simulink model "robot_stand"  (R2014b)
settings: Solver=ode45  StartTime=0.0  StopTime=10  FixedStep=1e-4  RelTol=1e-3
values from neighbouring files (symbols this model uses):
  robot_floor_friction_coeff = 0.6    [robot_init.m]
  robot_floor_position_gain = -1e5    (= -100000)    [robot_init.m]
  robot_floor_speed_gain = -1e3    (= -1000)    [robot_init.m]
  robot_gravity = [0 0 -9.80665]    [robot_init.m]
undefined symbols (not defined in the file or in its folder): CM730_acc_center, CM730_acc_gain, CM730_default, CM730_gyro_center, CM730_gyro_gain, CM730_sample_time, FSR_max, FSR_no_load, FSR_sample_time, FSR_scale, MX28_default, MX28_inertia, MX28_Te, X, Y, Z
libraries: sm_lib x158, fl_lib x128, nesl_utility x77
(part 3 of 6)

== system robot_stand/Left Leg/Left Hip Pitch (12) ==
  Inertia : sm_lib/Body Elements/Inertia  InertiaType=Custom  Mass=1  MassUnits=g  CenterOfMass=[0 0 0]  CenterOfMassUnits=m  MomentsOfInertia=[0 0 MX28_inertia]  MomentsOfInertiaUnits=kg*m^2  ProductsOfInertia=[0 0 0]  ProductsOfInertiaUnits=kg*m^2  BlockFunction=simmechanics.library.body_elements.inertia
  MX28 Command : DataStoreRead  DataStoreName=MX28_ID12  SampleTime=MX28_Te  DataStoreElements=MX28_ID12.CW_angle_limit#MX28_ID12.CCW_angle_limit#MX28_ID12.torque_enable#MX28_ID12.D_gain#MX28_ID12.I_gain#MX28_ID12.P_gain#MX28_ID12.goal_position#MX28_ID12.moving_speed#MX28_ID12.torque_limit
  MX28 State : DataStoreWrite  DataStoreName=MX28_ID12  DataStoreElements=MX28_ID12.present_position#MX28_ID12.present_speed#MX28_ID12.present_load#MX28_ID12.moving#MX28_ID12.pwm
  Model : ModelReference  ModelNameDialog=MX28.slx  SimulationMode=Normal  ModelReferenceVersion=1.66  CopyOfModelName=MX28.slx  DefaultDataLogging=on
  Position converter : nesl_utility/PS-Simulink Converter  PhysicalDomain=network_engine_domain  SubClassName=ps_output  LeftPortType=input  RightPortType=output  PseudoPeriodic=off  Frequencies=[]  Unit=rad  AffineConversion=off
  Revolute Joint : sm_lib/Joints/Revolute Joint  SenseConstraintForce=off  SenseConstraintForceX=off  SenseConstraintForceY=off  SenseConstraintForceZ=off  SenseConstraintTorque=off  SenseConstraintTorqueX=off  SenseConstraintTorqueY=off  SenseConstraintTorqueZ=off  SenseTotalForce=off  SenseTotalForceX=off  SenseTotalForceY=off  SenseTotalForceZ=off  SenseTotalTorque=off  SenseTotalTorqueX=off  SenseTotalTorqueY=off  SenseTotalTorqueZ=off  CompositeWrenchDir=FollowerOnBase  CompositeWrenchFrame=BaseFrame  EquilibriumPosition=0  EquilibriumPositionUnits=deg  SpringStiffness=0  SpringStiffnessUnits=N*m/deg  DampingCoefficient=MX28_lub_friction  DampingCoefficientUnits=N*m/(rad/s)  TorqueActuationMode=InputTorque  MotionActuationMode=ComputedMotion  SensePosition=on  SenseVelocity=on  SenseAcceleration=off  SenseTorqueForce=off  PositionTargetValue=MX28_init_position  PositionTargetValueUnits=rad  PositionTargetSpecify=on  PositionTargetPriority=High  VelocityTargetValue=MX28_init_speed  VelocityTargetValueUnits=rad/s  VelocityTargetSpecify=on  VelocityTargetPriority=High  BlockFunction=simmechanics.library.joints.revolute_joint
  Speed converter : nesl_utility/PS-Simulink Converter  PhysicalDomain=network_engine_domain  SubClassName=ps_output  LeftPortType=input  RightPortType=output  PseudoPeriodic=off  Frequencies=[]  Unit=rad/s  AffineConversion=off
  Torque converter : nesl_utility/Simulink-PS Converter  PhysicalDomain=network_engine_domain  SubClassName=ps_input  LeftPortType=input  RightPortType=output  PseudoPeriodic=off  Frequencies=[]  NoiseDistribution=none  NoiseParameters=[]  Unit=N*m  AffineConversion=off  InputFiltering=off  SimscapeFilterOrder=1  InputFilterTimeConstant=0.001  UdotUserProvided=1
  Base : PMIOPort  Port=1  Side=Left
  Axis : PMIOPort  Port=2  Side=Right
  wires:
  Model/4 -> MX28 State/3
  Model/2 -> MX28 State/1
  Model/5 -> MX28 State/4
  Model/3 -> MX28 State/2
  MX28 Command/3 -> Model/5
  MX28 Command/6 -> Model/8
  MX28 Command/4 -> Model/6
  MX28 Command/5 -> Model/7
  MX28 Command/7 -> Model/9
  MX28 Command/2 -> Model/4
  MX28 Command/1 -> Model/3
  Speed converter/1 -> Model/1
  Position converter/1 -> Model/2
  Model/1 -> Torque converter/1
  Model/6 -> MX28 State/5
  MX28 Command/8 -> Model/10
  MX28 Command/9 -> Model/11
  connections:
  Axis/RConn1 -- Revolute Joint/RConn1 -- Inertia/RConn1
  Revolute Joint/LConn1 -- Base/RConn1
  Revolute Joint/RConn3 -- Speed converter/LConn1
  Revolute Joint/RConn2 -- Position converter/LConn1
  Revolute Joint/LConn2 -- Torque converter/RConn1

== system robot_stand/Left Leg/Left Hip Roll ==
  Left Hip Roll Base to Left Hip Pitch Base : sm_lib/Frames and Transforms/Rigid Transform  TranslationMethod=Cartesian  TranslationLengthUnit=mm  TranslationStandardAxis=+Z  TranslationStandardOffset=0  TranslationCartesianOffset=[-23.9 0 19.1]  TranslationROffset=0  TranslationROffsetUnits=m  TranslationZOffset=0  TranslationZOffsetUnits=m  TranslationThetaOffset=0  TranslationThetaOffsetUnits=deg  RotationMethod=AlignedAxes  RotationAngleUnits=deg  RotationStandardAxis=+Z  RotationAngle=0  RotationArbitraryAxis=[0 0 1]  FollAlignAxisA=+Y  BaseAlignAxisA=+Y  FollAlignAxisB=+X  BaseAlignAxisB=+Z  RotationMatrix=[1 0 0; 0 1 0; 0 0 1]  BlockFunction=simmechanics.library.frames_transforms.rigid_transform
  Solid : sm_lib/Body Elements/Solid  InertiaType=Custom  Mass=166.79  MassUnits=g  CenterOfMass=[0.3 -11.21 1.04]  CenterOfMassUnits=mm  MomentsOfInertia=[11815 12217 6971]  MomentsOfInertiaUnits=g*mm^2  ProductsOfInertia=[4000 -134 178]  ProductsOfInertiaUnits=g*mm^2  DensityBased=on  Density=1000  DensityUnits=kg/(m^3)  GraphicType=FromGeometry  MarkerShape=Sphere  MarkerSize=10  MarkerSizeUnits=m  GraphicVisPropType=SimpleVisualProperties  GraphicDiffuseColor=[0.5 0.5 0.5]  GraphicSpecularColor=[0.5 0.5 0.5 1.0]  GraphicAmbientColor=[0.15 0.15 0.15 1.0]  GraphicEmissiveColor=[0.0 0.0 0.0 1.0]  GraphicShininess=75  GraphicOpacity=1.0  GeometryShape=FromFile  RectangleSize=[1 1]  RectangleSizeUnits=m  BrickDimensions=[1 1 1]  BrickDimensionUnits=mm  CylinderRadius=1  CylinderRadiusUnits=m  CylinderLength=1  CylinderLengthUnits=m  SphereRadius=1  SphereRadiusUnits=m  EllipsoidRadii=[1 1 1]  EllipsoidRadiiUnits=m  ExtrusionCrossSection=[1 1; -1 1; -1 -1; 1 -1]  ExtrusionCrossSectionUnits=m  ExtrusionLength=1  ExtrusionLengthUnits=m  PolygonNumSides=3  PolygonOuterRadius=1  PolygonOuterRadiusUnits=m  ExtGeomFileType=STL  ExtGeomFileName=D:\Ker Lann\systemes\darwin\kinematics\STL\Left_Hip2.STL  ExtGeomFileUnits=mm  RevolutionCrossSection=[1 1; 1 -1; 2 -1; 2 1]  RevolutionCrossSectionUnits=m  RevolutionExtent=Full  RevolutionAngle=180  RevolutionAngleUnits=deg  BlockFunction=simmechanics.library.body_elements.solid
  Left Hip Roll : PMIOPort  Port=1  Side=Left
  Left Hip Pitch : PMIOPort  Port=2  Side=Right
  connections:
  Left Hip Roll Base to Left Hip Pitch Base/LConn1 -- Solid/RConn1 -- Left Hip Roll/RConn1
  Left Hip Roll Base to Left Hip Pitch Base/RConn1 -- Left Hip Pitch/RConn1

== system robot_stand/Left Leg/Left Hip Roll (10) ==
  Inertia : sm_lib/Body Elements/Inertia  InertiaType=Custom  Mass=1  MassUnits=g  CenterOfMass=[0 0 0]  CenterOfMassUnits=m  MomentsOfInertia=[0 0 MX28_inertia]  MomentsOfInertiaUnits=kg*m^2  ProductsOfInertia=[0 0 0]  ProductsOfInertiaUnits=kg*m^2  BlockFunction=simmechanics.library.body_elements.inertia
  MX28 Command : DataStoreRead  DataStoreName=MX28_ID10  SampleTime=MX28_Te  DataStoreElements=MX28_ID10.CW_angle_limit#MX28_ID10.CCW_angle_limit#MX28_ID10.torque_enable#MX28_ID10.D_gain#MX28_ID10.I_gain#MX28_ID10.P_gain#MX28_ID10.goal_position#MX28_ID10.moving_speed#MX28_ID10.torque_limit
  MX28 State : DataStoreWrite  DataStoreName=MX28_ID10  DataStoreElements=MX28_ID10.present_position#MX28_ID10.present_speed#MX28_ID10.present_load#MX28_ID10.moving#MX28_ID10.pwm
  Model : ModelReference  ModelNameDialog=MX28.slx  SimulationMode=Normal  ModelReferenceVersion=1.66  CopyOfModelName=MX28.slx  DefaultDataLogging=on
  Position converter : nesl_utility/PS-Simulink Converter  PhysicalDomain=network_engine_domain  SubClassName=ps_output  LeftPortType=input  RightPortType=output  PseudoPeriodic=off  Frequencies=[]  Unit=rad  AffineConversion=off
  Revolute Joint : sm_lib/Joints/Revolute Joint  SenseConstraintForce=off  SenseConstraintForceX=off  SenseConstraintForceY=off  SenseConstraintForceZ=off  SenseConstraintTorque=off  SenseConstraintTorqueX=off  SenseConstraintTorqueY=off  SenseConstraintTorqueZ=off  SenseTotalForce=off  SenseTotalForceX=off  SenseTotalForceY=off  SenseTotalForceZ=off  SenseTotalTorque=off  SenseTotalTorqueX=off  SenseTotalTorqueY=off  SenseTotalTorqueZ=off  CompositeWrenchDir=FollowerOnBase  CompositeWrenchFrame=BaseFrame  EquilibriumPosition=0  EquilibriumPositionUnits=deg  SpringStiffness=0  SpringStiffnessUnits=N*m/deg  DampingCoefficient=MX28_lub_friction  DampingCoefficientUnits=N*m/(rad/s)  TorqueActuationMode=InputTorque  MotionActuationMode=ComputedMotion  SensePosition=on  SenseVelocity=on  SenseAcceleration=off  SenseTorqueForce=off  PositionTargetValue=MX28_init_position  PositionTargetValueUnits=rad  PositionTargetSpecify=on  PositionTargetPriority=High  VelocityTargetValue=MX28_init_speed  VelocityTargetValueUnits=rad/s  VelocityTargetSpecify=on  VelocityTargetPriority=High  BlockFunction=simmechanics.library.joints.revolute_joint
  Speed converter : nesl_utility/PS-Simulink Converter  PhysicalDomain=network_engine_domain  SubClassName=ps_output  LeftPortType=input  RightPortType=output  PseudoPeriodic=off  Frequencies=[]  Unit=rad/s  AffineConversion=off
  Torque converter : nesl_utility/Simulink-PS Converter  PhysicalDomain=network_engine_domain  SubClassName=ps_input  LeftPortType=input  RightPortType=output  PseudoPeriodic=off  Frequencies=[]  NoiseDistribution=none  NoiseParameters=[]  Unit=N*m  AffineConversion=off  InputFiltering=off  SimscapeFilterOrder=1  InputFilterTimeConstant=0.001  UdotUserProvided=1
  Base : PMIOPort  Port=1  Side=Left
  Axis : PMIOPort  Port=2  Side=Right
  wires:
  Model/4 -> MX28 State/3
  Model/2 -> MX28 State/1
  Model/5 -> MX28 State/4
  Model/3 -> MX28 State/2
  MX28 Command/3 -> Model/5
  MX28 Command/6 -> Model/8
  MX28 Command/4 -> Model/6
  MX28 Command/5 -> Model/7
  MX28 Command/7 -> Model/9
  MX28 Command/2 -> Model/4
  MX28 Command/1 -> Model/3
  Position converter/1 -> Model/2
  Speed converter/1 -> Model/1
  Model/1 -> Torque converter/1
  Model/6 -> MX28 State/5
  MX28 Command/8 -> Model/10
  MX28 Command/9 -> Model/11
  connections:
  Axis/RConn1 -- Revolute Joint/RConn1 -- Inertia/RConn1
  Revolute Joint/LConn1 -- Base/RConn1
  Revolute Joint/RConn3 -- Speed converter/LConn1
  Revolute Joint/RConn2 -- Position converter/LConn1
  Revolute Joint/LConn2 -- Torque converter/RConn1

== system robot_stand/Left Leg/Left Hip Yaw ==
  Left Hip Yaw Axis to Left Hip Roll Axis : sm_lib/Frames and Transforms/Rigid Transform  TranslationMethod=Cartesian  TranslationLengthUnit=mm  TranslationStandardAxis=+Z  TranslationStandardOffset=0  TranslationCartesianOffset=[24.85 0 28.35]  TranslationROffset=0  TranslationROffsetUnits=m  TranslationZOffset=0  TranslationZOffsetUnits=m  TranslationThetaOffset=0  TranslationThetaOffsetUnits=deg  RotationMethod=AlignedAxes  RotationAngleUnits=deg  RotationStandardAxis=+Z  RotationAngle=0  RotationArbitraryAxis=[0 0 1]  FollAlignAxisA=+Y  BaseAlignAxisA=+Z  FollAlignAxisB=+X  BaseAlignAxisB=-Y  RotationMatrix=[1 0 0; 0 1 0; 0 0 1]  BlockFunction=simmechanics.library.frames_transforms.rigid_transform
  Solid : sm_lib/Body Elements/Solid  InertiaType=Custom  Mass=34.1  MassUnits=g  CenterOfMass=[7.53 0 10.27]  CenterOfMassUnits=mm  MomentsOfInertia=[8263 18980 13482]  MomentsOfInertiaUnits=g*mm^2  ProductsOfInertia=[0 3667 0]  ProductsOfInertiaUnits=g*mm^2  DensityBased=on  Density=1000  DensityUnits=kg/(m^3)  GraphicType=FromGeometry  MarkerShape=Sphere  MarkerSize=10  MarkerSizeUnits=m  GraphicVisPropType=SimpleVisualProperties  GraphicDiffuseColor=[0.5 0.5 0.5]  GraphicSpecularColor=[0.5 0.5 0.5 1.0]  GraphicAmbientColor=[0.15 0.15 0.15 1.0]  GraphicEmissiveColor=[0.0 0.0 0.0 1.0]  GraphicShininess=75  GraphicOpacity=1.0  GeometryShape=FromFile  RectangleSize=[1 1]  RectangleSizeUnits=m  BrickDimensions=[1 1 1]  BrickDimensionUnits=mm  CylinderRadius=1  CylinderRadiusUnits=m  CylinderLength=1  CylinderLengthUnits=m  SphereRadius=1  SphereRadiusUnits=m  EllipsoidRadii=[1 1 1]  EllipsoidRadiiUnits=m  ExtrusionCrossSection=[1 1; -1 1; -1 -1; 1 -1]  ExtrusionCrossSectionUnits=m  ExtrusionLength=1  ExtrusionLengthUnits=m  PolygonNumSides=3  PolygonOuterRadius=1  PolygonOuterRadiusUnits=m  ExtGeomFileType=STL  ExtGeomFileName=D:\Ker Lann\systemes\darwin\kinematics\STL\Hip1.STL  ExtGeomFileUnits=mm  RevolutionCrossSection=[1 1; 1 -1; 2 -1; 2 1]  RevolutionCrossSectionUnits=m  RevolutionExtent=Full  RevolutionAngle=180  RevolutionAngleUnits=deg  BlockFunction=simmechanics.library.body_elements.solid
  Left Hip Yaw : PMIOPort  Port=1  Side=Left
  Left Hip Roll : PMIOPort  Port=2  Side=Right
  connections:
  Left Hip Yaw/RConn1 -- Solid/RConn1 -- Left Hip Yaw Axis to Left Hip Roll Axis/LConn1
  Left Hip Yaw Axis to Left Hip Roll Axis/RConn1 -- Left Hip Roll/RConn1

== system robot_stand/Left Leg/Left Hip Yaw (8) ==
  Inertia : sm_lib/Body Elements/Inertia  InertiaType=Custom  Mass=1  MassUnits=g  CenterOfMass=[0 0 0]  CenterOfMassUnits=m  MomentsOfInertia=[0 0 MX28_inertia]  MomentsOfInertiaUnits=kg*m^2  ProductsOfInertia=[0 0 0]  ProductsOfInertiaUnits=kg*m^2  BlockFunction=simmechanics.library.body_elements.inertia
  MX28 Command : DataStoreRead  DataStoreName=MX28_ID8  SampleTime=MX28_Te  DataStoreElements=MX28_ID8.CW_angle_limit#MX28_ID8.CCW_angle_limit#MX28_ID8.torque_enable#MX28_ID8.D_gain#MX28_ID8.I_gain#MX28_ID8.P_gain#MX28_ID8.goal_position#MX28_ID8.moving_speed#MX28_ID8.torque_limit
  MX28 State : DataStoreWrite  DataStoreName=MX28_ID8  DataStoreElements=MX28_ID8.present_position#MX28_ID8.present_speed#MX28_ID8.present_load#MX28_ID8.moving#MX28_ID8.pwm
  Model : ModelReference  ModelNameDialog=MX28.slx  SimulationMode=Normal  ModelReferenceVersion=1.66  CopyOfModelName=MX28.slx  DefaultDataLogging=on
  Position converter : nesl_utility/PS-Simulink Converter  PhysicalDomain=network_engine_domain  SubClassName=ps_output  LeftPortType=input  RightPortType=output  PseudoPeriodic=off  Frequencies=[]  Unit=rad  AffineConversion=off
  Revolute Joint : sm_lib/Joints/Revolute Joint  SenseConstraintForce=off  SenseConstraintForceX=off  SenseConstraintForceY=off  SenseConstraintForceZ=off  SenseConstraintTorque=off  SenseConstraintTorqueX=off  SenseConstraintTorqueY=off  SenseConstraintTorqueZ=off  SenseTotalForce=off  SenseTotalForceX=off  SenseTotalForceY=off  SenseTotalForceZ=off  SenseTotalTorque=off  SenseTotalTorqueX=off  SenseTotalTorqueY=off  SenseTotalTorqueZ=off  CompositeWrenchDir=FollowerOnBase  CompositeWrenchFrame=BaseFrame  EquilibriumPosition=0  EquilibriumPositionUnits=deg  SpringStiffness=0  SpringStiffnessUnits=N*m/deg  DampingCoefficient=MX28_lub_friction  DampingCoefficientUnits=N*m/(rad/s)  TorqueActuationMode=InputTorque  MotionActuationMode=ComputedMotion  SensePosition=on  SenseVelocity=on  SenseAcceleration=off  SenseTorqueForce=off  PositionTargetValue=MX28_init_position  PositionTargetValueUnits=rad  PositionTargetSpecify=on  PositionTargetPriority=High  VelocityTargetValue=MX28_init_speed  VelocityTargetValueUnits=rad/s  VelocityTargetSpecify=on  VelocityTargetPriority=High  BlockFunction=simmechanics.library.joints.revolute_joint
  Speed converter : nesl_utility/PS-Simulink Converter  PhysicalDomain=network_engine_domain  SubClassName=ps_output  LeftPortType=input  RightPortType=output  PseudoPeriodic=off  Frequencies=[]  Unit=rad/s  AffineConversion=off
  Torque converter : nesl_utility/Simulink-PS Converter  PhysicalDomain=network_engine_domain  SubClassName=ps_input  LeftPortType=input  RightPortType=output  PseudoPeriodic=off  Frequencies=[]  NoiseDistribution=none  NoiseParameters=[]  Unit=N*m  AffineConversion=off  InputFiltering=off  SimscapeFilterOrder=1  InputFilterTimeConstant=0.001  UdotUserProvided=1
  Base : PMIOPort  Port=1  Side=Left
  Axis : PMIOPort  Port=2  Side=Right
  wires:
  Model/4 -> MX28 State/3
  Model/2 -> MX28 State/1
  Model/5 -> MX28 State/4
  Model/3 -> MX28 State/2
  MX28 Command/3 -> Model/5
  MX28 Command/6 -> Model/8
  MX28 Command/4 -> Model/6
  MX28 Command/5 -> Model/7
  MX28 Command/7 -> Model/9
  MX28 Command/2 -> Model/4
  MX28 Command/1 -> Model/3
  Speed converter/1 -> Model/1
  Position converter/1 -> Model/2
  Model/1 -> Torque converter/1
  Model/6 -> MX28 State/5
  MX28 Command/8 -> Model/10
  MX28 Command/9 -> Model/11
  connections:
  Axis/RConn1 -- Revolute Joint/RConn1 -- Inertia/RConn1
  Revolute Joint/LConn1 -- Base/RConn1
  Revolute Joint/RConn3 -- Speed converter/LConn1
  Revolute Joint/RConn2 -- Position converter/LConn1
  Revolute Joint/LConn2 -- Torque converter/RConn1

== system robot_stand/Left Leg/Left Knee (14) ==
  Inertia : sm_lib/Body Elements/Inertia  InertiaType=Custom  Mass=1  MassUnits=g  CenterOfMass=[0 0 0]  CenterOfMassUnits=m  MomentsOfInertia=[0 0 MX28_inertia]  MomentsOfInertiaUnits=kg*m^2  ProductsOfInertia=[0 0 0]  ProductsOfInertiaUnits=kg*m^2  BlockFunction=simmechanics.library.body_elements.inertia
  MX28 Command : DataStoreRead  DataStoreName=MX28_ID14  SampleTime=MX28_Te  DataStoreElements=MX28_ID14.CW_angle_limit#MX28_ID14.CCW_angle_limit#MX28_ID14.torque_enable#MX28_ID14.D_gain#MX28_ID14.I_gain#MX28_ID14.P_gain#MX28_ID14.goal_position#MX28_ID14.moving_speed#MX28_ID14.torque_limit
  MX28 State : DataStoreWrite  DataStoreName=MX28_ID14  DataStoreElements=MX28_ID14.present_position#MX28_ID14.present_speed#MX28_ID14.present_load#MX28_ID14.moving#MX28_ID14.pwm
  Model : ModelReference  ModelNameDialog=MX28.slx  SimulationMode=Normal  ModelReferenceVersion=1.66  CopyOfModelName=MX28.slx  DefaultDataLogging=on
  Position converter : nesl_utility/PS-Simulink Converter  PhysicalDomain=network_engine_domain  SubClassName=ps_output  LeftPortType=input  RightPortType=output  PseudoPeriodic=off  Frequencies=[]  Unit=rad  AffineConversion=off
  Revolute Joint : sm_lib/Joints/Revolute Joint  SenseConstraintForce=off  SenseConstraintForceX=off  SenseConstraintForceY=off  SenseConstraintForceZ=off  SenseConstraintTorque=off  SenseConstraintTorqueX=off  SenseConstraintTorqueY=off  SenseConstraintTorqueZ=off  SenseTotalForce=off  SenseTotalForceX=off  SenseTotalForceY=off  SenseTotalForceZ=off  SenseTotalTorque=off  SenseTotalTorqueX=off  SenseTotalTorqueY=off  SenseTotalTorqueZ=off  CompositeWrenchDir=FollowerOnBase  CompositeWrenchFrame=BaseFrame  EquilibriumPosition=0  EquilibriumPositionUnits=deg  SpringStiffness=0  SpringStiffnessUnits=N*m/deg  DampingCoefficient=MX28_lub_friction  DampingCoefficientUnits=N*m/(rad/s)  TorqueActuationMode=InputTorque  MotionActuationMode=ComputedMotion  SensePosition=on  SenseVelocity=on  SenseAcceleration=off  SenseTorqueForce=off  PositionTargetValue=MX28_init_position  PositionTargetValueUnits=rad  PositionTargetSpecify=on  PositionTargetPriority=High  VelocityTargetValue=MX28_init_speed  VelocityTargetValueUnits=rad/s  VelocityTargetSpecify=on  VelocityTargetPriority=High  BlockFunction=simmechanics.library.joints.revolute_joint
  Speed converter : nesl_utility/PS-Simulink Converter  PhysicalDomain=network_engine_domain  SubClassName=ps_output  LeftPortType=input  RightPortType=output  PseudoPeriodic=off  Frequencies=[]  Unit=rad/s  AffineConversion=off
  Torque converter : nesl_utility/Simulink-PS Converter  PhysicalDomain=network_engine_domain  SubClassName=ps_input  LeftPortType=input  RightPortType=output  PseudoPeriodic=off  Frequencies=[]  NoiseDistribution=none  NoiseParameters=[]  Unit=N*m  AffineConversion=off  InputFiltering=off  SimscapeFilterOrder=1  InputFilterTimeConstant=0.001  UdotUserProvided=1
  Base : PMIOPort  Port=1  Side=Left
  Axis : PMIOPort  Port=2  Side=Right
  wires:
  Model/4 -> MX28 State/3
  Model/2 -> MX28 State/1
  Model/5 -> MX28 State/4
  Model/3 -> MX28 State/2
  MX28 Command/3 -> Model/5
  MX28 Command/6 -> Model/8
  MX28 Command/4 -> Model/6
  MX28 Command/5 -> Model/7
  MX28 Command/7 -> Model/9
  MX28 Command/2 -> Model/4
  MX28 Command/1 -> Model/3
  Speed converter/1 -> Model/1
  Position converter/1 -> Model/2
  Model/1 -> Torque converter/1
  Model/6 -> MX28 State/5
  MX28 Command/8 -> Model/10
  MX28 Command/9 -> Model/11
  connections:
  Axis/RConn1 -- Revolute Joint/RConn1 -- Inertia/RConn1
  Revolute Joint/LConn1 -- Base/RConn1
  Revolute Joint/RConn3 -- Speed converter/LConn1
  Revolute Joint/RConn2 -- Position converter/LConn1
  Revolute Joint/LConn2 -- Torque converter/RConn1

== system robot_stand/Left Leg/Left Lower Leg ==
  Left Lower Leg Axis to Left Ankle  Axis : sm_lib/Frames and Transforms/Rigid Transform  TranslationMethod=Cartesian  TranslationLengthUnit=mm  TranslationStandardAxis=+Z  TranslationStandardOffset=0  TranslationCartesianOffset=[0 -93 0]  TranslationROffset=0  TranslationROffsetUnits=m  TranslationZOffset=0  TranslationZOffsetUnits=m  TranslationThetaOffset=0  TranslationThetaOffsetUnits=deg  RotationMethod=None  RotationAngleUnits=deg  RotationStandardAxis=+Z  RotationAngle=0  RotationArbitraryAxis=[0 0 1]  FollAlignAxisA=+X  BaseAlignAxisA=+Y  FollAlignAxisB=+Y  BaseAlignAxisB=+Z  RotationMatrix=[1 0 0; 0 1 0; 0 0 1]  BlockFunction=simmechanics.library.frames_transforms.rigid_transform
  Solid : sm_lib/Body Elements/Solid  InertiaType=Custom  Mass=76.54  MassUnits=g  CenterOfMass=[6.06 -39.15 -19.66]  CenterOfMassUnits=mm  MomentsOfInertia=[128593 47766 107886]  MomentsOfInertiaUnits=g*mm^2  ProductsOfInertia=[-2242 -1853 13175]  ProductsOfInertiaUnits=g*mm^2  DensityBased=on  Density=1000  DensityUnits=kg/(m^3)  GraphicType=FromGeometry  MarkerShape=Sphere  MarkerSize=10  MarkerSizeUnits=m  GraphicVisPropType=SimpleVisualProperties  GraphicDiffuseColor=[0.5 0.5 0.5]  GraphicSpecularColor=[0.5 0.5 0.5 1.0]  GraphicAmbientColor=[0.15 0.15 0.15 1.0]  GraphicEmissiveColor=[0.0 0.0 0.0 1.0]  GraphicShininess=75  GraphicOpacity=1.0  GeometryShape=FromFile  RectangleSize=[1 1]  RectangleSizeUnits=m  BrickDimensions=[1 1 1]  BrickDimensionUnits=m  CylinderRadius=1  CylinderRadiusUnits=m  CylinderLength=1  CylinderLengthUnits=m  SphereRadius=1  SphereRadiusUnits=m  EllipsoidRadii=[1 1 1]  EllipsoidRadiiUnits=m  ExtrusionCrossSection=[1 1; -1 1; -1 -1; 1 -1]  ExtrusionCrossSectionUnits=m  ExtrusionLength=1  ExtrusionLengthUnits=m  PolygonNumSides=3  PolygonOuterRadius=1  PolygonOuterRadiusUnits=m  ExtGeomFileType=STL  ExtGeomFileName=D:\Ker Lann\systemes\darwin\kinematics\STL\Left_Lower_Leg.STL  ExtGeomFileUnits=mm  RevolutionCrossSection=[1 1; 1 -1; 2 -1; 2 1]  RevolutionCrossSectionUnits=m  RevolutionExtent=Full  RevolutionAngle=180  RevolutionAngleUnits=deg  BlockFunction=simmechanics.library.body_elements.solid
  Left Knee : PMIOPort  Port=1  Side=Left
  Left Ankle Pitch : PMIOPort  Port=2  Side=Right
  connections:
  Solid/RConn1 -- Left Lower Leg Axis to Left Ankle  Axis/LConn1 -- Left Knee/RConn1
  Left Ankle Pitch/RConn1 -- Left Lower Leg Axis to Left Ankle  Axis/RConn1

== system robot_stand/Left Leg/Left Thigh ==
  Left Hip Pitch Axis to Left Lower Leg Base : sm_lib/Frames and Transforms/Rigid Transform  TranslationMethod=Cartesian  TranslationLengthUnit=mm  TranslationStandardAxis=+Z  TranslationStandardOffset=0  TranslationCartesianOffset=[0 93 0.25]  TranslationROffset=0  TranslationROffsetUnits=m  TranslationZOffset=0  TranslationZOffsetUnits=m  TranslationThetaOffset=0  TranslationThetaOffsetUnits=deg  RotationMethod=None  RotationAngleUnits=deg  RotationStandardAxis=+Z  RotationAngle=0  RotationArbitraryAxis=[0 0 1]  FollAlignAxisA=+X  BaseAlignAxisA=+Y  FollAlignAxisB=+Y  BaseAlignAxisB=+Z  RotationMatrix=[1 0 0; 0 1 0; 0 0 1]  BlockFunction=simmechanics.library.frames_transforms.rigid_transform
  Solid : sm_lib/Body Elements/Solid  InertiaType=Custom  Mass=120.35  MassUnits=g  CenterOfMass=[-0.84 62.83 -22.82]  CenterOfMassUnits=mm  MomentsOfInertia=[55246 22028 41171]  MomentsOfInertiaUnits=g*mm^2  ProductsOfInertia=[-6444 246 -1518]  ProductsOfInertiaUnits=g*mm^2  DensityBased=on  Density=1000  DensityUnits=kg/(m^3)  GraphicType=FromGeometry  MarkerShape=Sphere  MarkerSize=10  MarkerSizeUnits=m  GraphicVisPropType=SimpleVisualProperties  GraphicDiffuseColor=[0.5 0.5 0.5]  GraphicSpecularColor=[0.5 0.5 0.5 1.0]  GraphicAmbientColor=[0.15 0.15 0.15 1.0]  GraphicEmissiveColor=[0.0 0.0 0.0 1.0]  GraphicShininess=75  GraphicOpacity=1.0  GeometryShape=FromFile  RectangleSize=[1 1]  RectangleSizeUnits=m  BrickDimensions=[1 1 1]  BrickDimensionUnits=m  CylinderRadius=1  CylinderRadiusUnits=m  CylinderLength=1  CylinderLengthUnits=m  SphereRadius=1  SphereRadiusUnits=m  EllipsoidRadii=[1 1 1]  EllipsoidRadiiUnits=m  ExtrusionCrossSection=[1 1; -1 1; -1 -1; 1 -1]  ExtrusionCrossSectionUnits=m  ExtrusionLength=1  ExtrusionLengthUnits=m  PolygonNumSides=3  PolygonOuterRadius=1  PolygonOuterRadiusUnits=m  ExtGeomFileType=STL  ExtGeomFileName=D:\Ker Lann\systemes\darwin\kinematics\STL\Left_Thigh.STL  ExtGeomFileUnits=mm  RevolutionCrossSection=[1 1; 1 -1; 2 -1; 2 1]  RevolutionCrossSectionUnits=m  RevolutionExtent=Full  RevolutionAngle=180  RevolutionAngleUnits=deg  BlockFunction=simmechanics.library.body_elements.solid
  Left Hip Pitch : PMIOPort  Port=1  Side=Left
  Left Knee : PMIOPort  Port=2  Side=Right
  connections:
  Solid/RConn1 -- Left Hip Pitch Axis to Left Lower Leg Base/LConn1 -- Left Hip Pitch/RConn1
  Left Knee/RConn1 -- Left Hip Pitch Axis to Left Lower Leg Base/RConn1

== system robot_stand/Right Arm/Right Elbow (5) ==
  Inertia : sm_lib/Body Elements/Inertia  InertiaType=Custom  Mass=1  MassUnits=g  CenterOfMass=[0 0 0]  CenterOfMassUnits=m  MomentsOfInertia=[0 0 MX28_inertia]  MomentsOfInertiaUnits=kg*m^2  ProductsOfInertia=[0 0 0]  ProductsOfInertiaUnits=kg*m^2  BlockFunction=simmechanics.library.body_elements.inertia
  MX28 Command : DataStoreRead  DataStoreName=MX28_ID5  SampleTime=MX28_Te  DataStoreElements=MX28_ID5.CW_angle_limit#MX28_ID5.CCW_angle_limit#MX28_ID5.torque_enable#MX28_ID5.D_gain#MX28_ID5.I_gain#MX28_ID5.P_gain#MX28_ID5.goal_position#MX28_ID5.moving_speed#MX28_ID5.torque_limit
  MX28 State : DataStoreWrite  DataStoreName=MX28_ID5  DataStoreElements=MX28_ID5.present_position#MX28_ID5.present_speed#MX28_ID5.present_load#MX28_ID5.moving#MX28_ID5.pwm
  Model : ModelReference  ModelNameDialog=MX28.slx  SimulationMode=Normal  ModelReferenceVersion=1.66  CopyOfModelName=MX28.slx  DefaultDataLogging=on
  Position converter : nesl_utility/PS-Simulink Converter  PhysicalDomain=network_engine_domain  SubClassName=ps_output  LeftPortType=input  RightPortType=output  PseudoPeriodic=off  Frequencies=[]  Unit=rad  AffineConversion=off
  Revolute Joint : sm_lib/Joints/Revolute Joint  SenseConstraintForce=off  SenseConstraintForceX=off  SenseConstraintForceY=off  SenseConstraintForceZ=off  SenseConstraintTorque=off  SenseConstraintTorqueX=off  SenseConstraintTorqueY=off  SenseConstraintTorqueZ=off  SenseTotalForce=off  SenseTotalForceX=off  SenseTotalForceY=off  SenseTotalForceZ=off  SenseTotalTorque=off  SenseTotalTorqueX=off  SenseTotalTorqueY=off  SenseTotalTorqueZ=off  CompositeWrenchDir=FollowerOnBase  CompositeWrenchFrame=BaseFrame  EquilibriumPosition=0  EquilibriumPositionUnits=deg  SpringStiffness=0  SpringStiffnessUnits=N*m/deg  DampingCoefficient=MX28_lub_friction  DampingCoefficientUnits=N*m/(rad/s)  TorqueActuationMode=InputTorque  MotionActuationMode=ComputedMotion  SensePosition=on  SenseVelocity=on  SenseAcceleration=off  SenseTorqueForce=off  PositionTargetValue=MX28_init_position  PositionTargetValueUnits=rad  PositionTargetSpecify=on  PositionTargetPriority=High  VelocityTargetValue=MX28_init_speed  VelocityTargetValueUnits=rad/s  VelocityTargetSpecify=on  VelocityTargetPriority=High  BlockFunction=simmechanics.library.joints.revolute_joint
  Speed converter : nesl_utility/PS-Simulink Converter  PhysicalDomain=network_engine_domain  SubClassName=ps_output  LeftPortType=input  RightPortType=output  PseudoPeriodic=off  Frequencies=[]  Unit=rad/s  AffineConversion=off
  Torque converter : nesl_utility/Simulink-PS Converter  PhysicalDomain=network_engine_domain  SubClassName=ps_input  LeftPortType=input  RightPortType=output  PseudoPeriodic=off  Frequencies=[]  NoiseDistribution=none  NoiseParameters=[]  Unit=N*m  AffineConversion=off  InputFiltering=off  SimscapeFilterOrder=1  InputFilterTimeConstant=0.001  UdotUserProvided=1
  Base : PMIOPort  Port=1  Side=Left
  Axis : PMIOPort  Port=2  Side=Right
  wires:
  Model/4 -> MX28 State/3
  Model/2 -> MX28 State/1
  Model/5 -> MX28 State/4
  Model/3 -> MX28 State/2
  MX28 Command/3 -> Model/5
  MX28 Command/6 -> Model/8
  MX28 Command/4 -> Model/6
  MX28 Command/5 -> Model/7
  MX28 Command/7 -> Model/9
  MX28 Command/2 -> Model/4
  MX28 Command/1 -> Model/3
  Speed converter/1 -> Model/1
  Position converter/1 -> Model/2
  Model/1 -> Torque converter/1
  Model/6 -> MX28 State/5
  MX28 Command/8 -> Model/10
  MX28 Command/9 -> Model/11
  connections:
  Axis/RConn1 -- Revolute Joint/RConn1 -- Inertia/RConn1
  Revolute Joint/RConn3 -- Speed converter/LConn1
  Revolute Joint/RConn2 -- Position converter/LConn1
  Revolute Joint/LConn2 -- Torque converter/RConn1
  Revolute Joint/LConn1 -- Base/RConn1

== system robot_stand/Right Arm/Right Forearm ==
  Solid : sm_lib/Body Elements/Solid  InertiaType=Custom  Mass=62.79  MassUnits=g  CenterOfMass=[12.76 43.34 -15.75]  CenterOfMassUnits=mm  MomentsOfInertia=[94510 21923 95153]  MomentsOfInertiaUnits=g*mm^2  ProductsOfInertia=[1625 -659.23 8489]  ProductsOfInertiaUnits=g*mm^2  DensityBased=on  Density=1000  DensityUnits=kg/(m^3)  GraphicType=FromGeometry  MarkerShape=Sphere  MarkerSize=10  MarkerSizeUnits=m  GraphicVisPropType=SimpleVisualProperties  GraphicDiffuseColor=[0.5 0.5 0.5]  GraphicSpecularColor=[0.5 0.5 0.5 1.0]  GraphicAmbientColor=[0.15 0.15 0.15 1.0]  GraphicEmissiveColor=[0.0 0.0 0.0 1.0]  GraphicShininess=75  GraphicOpacity=1.0  GeometryShape=FromFile  RectangleSize=[1 1]  RectangleSizeUnits=m  BrickDimensions=[1 1 1]  BrickDimensionUnits=m  CylinderRadius=1  CylinderRadiusUnits=m  CylinderLength=1  CylinderLengthUnits=m  SphereRadius=1  SphereRadiusUnits=m  EllipsoidRadii=[1 1 1]  EllipsoidRadiiUnits=m  ExtrusionCrossSection=[1 1; -1 1; -1 -1; 1 -1]  ExtrusionCrossSectionUnits=m  ExtrusionLength=1  ExtrusionLengthUnits=m  PolygonNumSides=3  PolygonOuterRadius=1  PolygonOuterRadiusUnits=m  ExtGeomFileType=STL  ExtGeomFileName=D:\Ker Lann\systemes\darwin\kinematics\STL\Right_Forearm.STL  ExtGeomFileUnits=mm  RevolutionCrossSection=[1 1; 1 -1; 2 -1; 2 1]  RevolutionCrossSectionUnits=m  RevolutionExtent=Full  RevolutionAngle=180  RevolutionAngleUnits=deg  BlockFunction=simmechanics.library.body_elements.solid
  Right Elbow : PMIOPort  Port=1  Side=Left
  connections:
  Right Elbow/RConn1 -- Solid/RConn1

== system robot_stand/Right Arm/Right Shoulder ==
  Right Shoulder Axis to Right Arm Base 1/2 : sm_lib/Frames and Transforms/Rigid Transform  TranslationMethod=Cartesian  TranslationLengthUnit=mm  TranslationStandardAxis=+Z  TranslationStandardOffset=0  TranslationCartesianOffset=[-23.65 16 21.35]  TranslationROffset=0  TranslationROffsetUnits=m  TranslationZOffset=0  TranslationZOffsetUnits=m  TranslationThetaOffset=0  TranslationThetaOffsetUnits=deg  RotationMethod=StandardAxis  RotationAngleUnits=deg  RotationStandardAxis=+Y  RotationAngle=270  RotationArbitraryAxis=[0 0 1]  FollAlignAxisA=+X  BaseAlignAxisA=+Y  FollAlignAxisB=+Y  BaseAlignAxisB=+Z  RotationMatrix=[1 0 0; 0 1 0; 0 0 1]  BlockFunction=simmechanics.library.frames_transforms.rigid_transform
  Right Shoulder Axis to Right Arm Base 2/2 : sm_lib/Frames and Transforms/Rigid Transform  TranslationMethod=None  TranslationLengthUnit=mm  TranslationStandardAxis=+Z  TranslationStandardOffset=0  TranslationCartesianOffset=[-23.65 16 21.35]  TranslationROffset=0  TranslationROffsetUnits=m  TranslationZOffset=0  TranslationZOffsetUnits=m  TranslationThetaOffset=0  TranslationThetaOffsetUnits=deg  RotationMethod=StandardAxis  RotationAngleUnits=deg  RotationStandardAxis=+Z  RotationAngle=+135  RotationArbitraryAxis=[0 0 1]  FollAlignAxisA=+X  BaseAlignAxisA=+Y  FollAlignAxisB=+Y  BaseAlignAxisB=+Z  RotationMatrix=[1 0 0; 0 1 0; 0 0 1]  BlockFunction=simmechanics.library.frames_transforms.rigid_transform
  Solid : sm_lib/Body Elements/Solid  InertiaType=Custom  Mass=34.03  MassUnits=g  CenterOfMass=[-4.16 5.98 7.64]  CenterOfMassUnits=mm  MomentsOfInertia=[7413 12768 11409]  MomentsOfInertiaUnits=g*mm^2  ProductsOfInertia=[2455 -1943 -1420]  ProductsOfInertiaUnits=g*mm^2  DensityBased=on  Density=1000  DensityUnits=kg/(m^3)  GraphicType=FromGeometry  MarkerShape=Sphere  MarkerSize=10  MarkerSizeUnits=m  GraphicVisPropType=SimpleVisualProperties  GraphicDiffuseColor=[0.5 0.5 0.5]  GraphicSpecularColor=[0.5 0.5 0.5 1.0]  GraphicAmbientColor=[0.15 0.15 0.15 1.0]  GraphicEmissiveColor=[0.0 0.0 0.0 1.0]  GraphicShininess=75  GraphicOpacity=1.0  GeometryShape=FromFile  RectangleSize=[1 1]  RectangleSizeUnits=m  BrickDimensions=[1 1 1]  BrickDimensionUnits=m  CylinderRadius=1  CylinderRadiusUnits=m  CylinderLength=1  CylinderLengthUnits=m  SphereRadius=1  SphereRadiusUnits=m  EllipsoidRadii=[1 1 1]  EllipsoidRadiiUnits=m  ExtrusionCrossSection=[1 1; -1 1; -1 -1; 1 -1]  ExtrusionCrossSectionUnits=m  ExtrusionLength=1  ExtrusionLengthUnits=m  PolygonNumSides=3  PolygonOuterRadius=1  PolygonOuterRadiusUnits=m  ExtGeomFileType=STL  ExtGeomFileName=D:\Ker Lann\systemes\darwin\kinematics\STL\Right_shoulder.STL  ExtGeomFileUnits=mm  RevolutionCrossSection=[1 1; 1 -1; 2 -1; 2 1]  RevolutionCrossSectionUnits=m  RevolutionExtent=Full  RevolutionAngle=180  RevolutionAngleUnits=deg  BlockFunction=simmechanics.library.body_elements.solid
  Right Shoulder Pitch : PMIOPort  Port=1  Side=Left
  Right Shoulder Roll : PMIOPort  Port=2  Side=Right
  connections:
  Solid/RConn1 -- Right Shoulder Axis to Right Arm Base 1/2/LConn1 -- Right Shoulder Pitch/RConn1
  Right Shoulder Axis to Right Arm Base 2/2/RConn1 -- Right Shoulder Roll/RConn1
  Right Shoulder Axis to Right Arm Base 1/2/RConn1 -- Right Shoulder Axis to Right Arm Base 2/2/LConn1

== system robot_stand/Right Arm/Right Shoulder Pitch (1) ==
  Inertia : sm_lib/Body Elements/Inertia  InertiaType=Custom  Mass=1  MassUnits=g  CenterOfMass=[0 0 0]  CenterOfMassUnits=m  MomentsOfInertia=[0 0 MX28_inertia]  MomentsOfInertiaUnits=kg*m^2  ProductsOfInertia=[0 0 0]  ProductsOfInertiaUnits=kg*m^2  BlockFunction=simmechanics.library.body_elements.inertia
  MX28 Command : DataStoreRead  DataStoreName=MX28_ID1  SampleTime=MX28_Te  DataStoreElements=MX28_ID1.CW_angle_limit#MX28_ID1.CCW_angle_limit#MX28_ID1.torque_enable#MX28_ID1.D_gain#MX28_ID1.I_gain#MX28_ID1.P_gain#MX28_ID1.goal_position#MX28_ID1.moving_speed#MX28_ID1.torque_limit
  MX28 State : DataStoreWrite  DataStoreName=MX28_ID1  DataStoreElements=MX28_ID1.present_position#MX28_ID1.present_speed#MX28_ID1.present_load#MX28_ID1.moving#MX28_ID1.pwm
  Model : ModelReference  ModelNameDialog=MX28.slx  SimulationMode=Normal  ModelReferenceVersion=1.66  CopyOfModelName=MX28.slx  DefaultDataLogging=on
  Position converter : nesl_utility/PS-Simulink Converter  PhysicalDomain=network_engine_domain  SubClassName=ps_output  LeftPortType=input  RightPortType=output  PseudoPeriodic=off  Frequencies=[]  Unit=rad  AffineConversion=off
  Revolute Joint : sm_lib/Joints/Revolute Joint  SenseConstraintForce=off  SenseConstraintForceX=off  SenseConstraintForceY=off  SenseConstraintForceZ=off  SenseConstraintTorque=off  SenseConstraintTorqueX=off  SenseConstraintTorqueY=off  SenseConstraintTorqueZ=off  SenseTotalForce=off  SenseTotalForceX=off  SenseTotalForceY=off  SenseTotalForceZ=off  SenseTotalTorque=off  SenseTotalTorqueX=off  SenseTotalTorqueY=off  SenseTotalTorqueZ=off  CompositeWrenchDir=FollowerOnBase  CompositeWrenchFrame=BaseFrame  EquilibriumPosition=0  EquilibriumPositionUnits=deg  SpringStiffness=0  SpringStiffnessUnits=N*m/deg  DampingCoefficient=MX28_lub_friction  DampingCoefficientUnits=N*m/(rad/s)  TorqueActuationMode=InputTorque  MotionActuationMode=ComputedMotion  SensePosition=on  SenseVelocity=on  SenseAcceleration=off  SenseTorqueForce=off  PositionTargetValue=MX28_init_position  PositionTargetValueUnits=rad  PositionTargetSpecify=on  PositionTargetPriority=High  VelocityTargetValue=MX28_init_speed  VelocityTargetValueUnits=rad/s  VelocityTargetSpecify=on  VelocityTargetPriority=High  BlockFunction=simmechanics.library.joints.revolute_joint
  Speed converter : nesl_utility/PS-Simulink Converter  PhysicalDomain=network_engine_domain  SubClassName=ps_output  LeftPortType=input  RightPortType=output  PseudoPeriodic=off  Frequencies=[]  Unit=rad/s  AffineConversion=off
  Torque converter : nesl_utility/Simulink-PS Converter  PhysicalDomain=network_engine_domain  SubClassName=ps_input  LeftPortType=input  RightPortType=output  PseudoPeriodic=off  Frequencies=[]  NoiseDistribution=none  NoiseParameters=[]  Unit=N*m  AffineConversion=off  InputFiltering=off  SimscapeFilterOrder=1  InputFilterTimeConstant=0.001  UdotUserProvided=1
  Base : PMIOPort  Port=1  Side=Left
  Axis : PMIOPort  Port=2  Side=Right
  wires:
  Model/4 -> MX28 State/3
  Model/2 -> MX28 State/1
  Model/5 -> MX28 State/4
  Model/3 -> MX28 State/2
  MX28 Command/3 -> Model/5
  MX28 Command/6 -> Model/8
  MX28 Command/4 -> Model/6
  MX28 Command/5 -> Model/7
  MX28 Command/7 -> Model/9
  MX28 Command/2 -> Model/4
  MX28 Command/1 -> Model/3
  Speed converter/1 -> Model/1
  Position converter/1 -> Model/2
  Model/1 -> Torque converter/1
  Model/6 -> MX28 State/5
  MX28 Command/8 -> Model/10
  MX28 Command/9 -> Model/11
  connections:
  Axis/RConn1 -- Revolute Joint/RConn1 -- Inertia/RConn1
  Revolute Joint/LConn1 -- Base/RConn1
  Revolute Joint/RConn3 -- Speed converter/LConn1
  Revolute Joint/RConn2 -- Position converter/LConn1
  Revolute Joint/LConn2 -- Torque converter/RConn1

== system robot_stand/Right Arm/Right Shoulder Roll (3) ==
  Inertia : sm_lib/Body Elements/Inertia  InertiaType=Custom  Mass=1  MassUnits=g  CenterOfMass=[0 0 0]  CenterOfMassUnits=m  MomentsOfInertia=[0 0 MX28_inertia]  MomentsOfInertiaUnits=kg*m^2  ProductsOfInertia=[0 0 0]  ProductsOfInertiaUnits=kg*m^2  BlockFunction=simmechanics.library.body_elements.inertia
  MX28 Command : DataStoreRead  DataStoreName=MX28_ID3  SampleTime=MX28_Te  DataStoreElements=MX28_ID3.CW_angle_limit#MX28_ID3.CCW_angle_limit#MX28_ID3.torque_enable#MX28_ID3.D_gain#MX28_ID3.I_gain#MX28_ID3.P_gain#MX28_ID3.goal_position#MX28_ID3.moving_speed#MX28_ID3.torque_limit
  MX28 State : DataStoreWrite  DataStoreName=MX28_ID3  DataStoreElements=MX28_ID3.present_position#MX28_ID3.present_speed#MX28_ID3.present_load#MX28_ID3.moving#MX28_ID3.pwm
  Model : ModelReference  ModelNameDialog=MX28.slx  SimulationMode=Normal  ModelReferenceVersion=1.66  CopyOfModelName=MX28.slx  DefaultDataLogging=on
  Position converter : nesl_utility/PS-Simulink Converter  PhysicalDomain=network_engine_domain  SubClassName=ps_output  LeftPortType=input  RightPortType=output  PseudoPeriodic=off  Frequencies=[]  Unit=rad  AffineConversion=off
  Revolute Joint : sm_lib/Joints/Revolute Joint  SenseConstraintForce=off  SenseConstraintForceX=off  SenseConstraintForceY=off  SenseConstraintForceZ=off  SenseConstraintTorque=off  SenseConstraintTorqueX=off  SenseConstraintTorqueY=off  SenseConstraintTorqueZ=off  SenseTotalForce=off  SenseTotalForceX=off  SenseTotalForceY=off  SenseTotalForceZ=off  SenseTotalTorque=off  SenseTotalTorqueX=off  SenseTotalTorqueY=off  SenseTotalTorqueZ=off  CompositeWrenchDir=FollowerOnBase  CompositeWrenchFrame=BaseFrame  EquilibriumPosition=0  EquilibriumPositionUnits=deg  SpringStiffness=0  SpringStiffnessUnits=N*m/deg  DampingCoefficient=MX28_lub_friction  DampingCoefficientUnits=N*m/(rad/s)  TorqueActuationMode=InputTorque  MotionActuationMode=ComputedMotion  SensePosition=on  SenseVelocity=on  SenseAcceleration=off  SenseTorqueForce=off  PositionTargetValue=MX28_init_position  PositionTargetValueUnits=rad  PositionTargetSpecify=on  PositionTargetPriority=High  VelocityTargetValue=MX28_init_speed  VelocityTargetValueUnits=rad/s  VelocityTargetSpecify=on  VelocityTargetPriority=High  BlockFunction=simmechanics.library.joints.revolute_joint
  Speed converter : nesl_utility/PS-Simulink Converter  PhysicalDomain=network_engine_domain  SubClassName=ps_output  LeftPortType=input  RightPortType=output  PseudoPeriodic=off  Frequencies=[]  Unit=rad/s  AffineConversion=off
  Torque converter : nesl_utility/Simulink-PS Converter  PhysicalDomain=network_engine_domain  SubClassName=ps_input  LeftPortType=input  RightPortType=output  PseudoPeriodic=off  Frequencies=[]  NoiseDistribution=none  NoiseParameters=[]  Unit=N*m  AffineConversion=off  InputFiltering=off  SimscapeFilterOrder=1  InputFilterTimeConstant=0.001  UdotUserProvided=1
  Base : PMIOPort  Port=1  Side=Left
  Axis : PMIOPort  Port=2  Side=Right
  wires:
  Model/4 -> MX28 State/3
  Model/2 -> MX28 State/1
  Model/5 -> MX28 State/4
  Model/3 -> MX28 State/2
  MX28 Command/3 -> Model/5
  MX28 Command/6 -> Model/8
  MX28 Command/4 -> Model/6
  MX28 Command/5 -> Model/7
  MX28 Command/7 -> Model/9
  MX28 Command/2 -> Model/4
  MX28 Command/1 -> Model/3
  Speed converter/1 -> Model/1
  Position converter/1 -> Model/2
  Model/1 -> Torque converter/1
  Model/6 -> MX28 State/5
  MX28 Command/8 -> Model/10
  MX28 Command/9 -> Model/11
  connections:
  Axis/RConn1 -- Revolute Joint/RConn1 -- Inertia/RConn1
  Revolute Joint/RConn3 -- Speed converter/LConn1
  Revolute Joint/RConn2 -- Position converter/LConn1
  Revolute Joint/LConn2 -- Torque converter/RConn1
  Revolute Joint/LConn1 -- Base/RConn1

== system robot_stand/Right Arm/Right Upper Arm ==
  Right Arm Axis to Right Forearm Base : sm_lib/Frames and Transforms/Rigid Transform  TranslationMethod=Cartesian  TranslationLengthUnit=mm  TranslationStandardAxis=+Z  TranslationStandardOffset=0  TranslationCartesianOffset=[23.9 60 -7.9]  TranslationROffset=0  TranslationROffsetUnits=m  TranslationZOffset=0  TranslationZOffsetUnits=m  TranslationThetaOffset=0  TranslationThetaOffsetUnits=deg  RotationMethod=AlignedAxes  RotationAngleUnits=deg  RotationStandardAxis=+Z  RotationAngle=0  RotationArbitraryAxis=[0 0 1]  FollAlignAxisA=+X  BaseAlignAxisA=-Y  FollAlignAxisB=+Z  BaseAlignAxisB=+X  RotationMatrix=[1 0 0; 0 1 0; 0 0 1]  BlockFunction=simmechanics.library.frames_transforms.rigid_transform
  Solid : sm_lib/Body Elements/Solid  InertiaType=Custom  Mass=164.27  MassUnits=g  CenterOfMass=[0.09 35.32 -22.36]  CenterOfMassUnits=mm  MomentsOfInertia=[10985 7003 10316]  MomentsOfInertiaUnits=g*mm^2  ProductsOfInertia=[1167 -369 -1558]  ProductsOfInertiaUnits=g*mm^2  DensityBased=on  Density=1000  DensityUnits=kg/(m^3)  GraphicType=FromGeometry  MarkerShape=Sphere  MarkerSize=10  MarkerSizeUnits=m  GraphicVisPropType=SimpleVisualProperties  GraphicDiffuseColor=[0.5 0.5 0.5]  GraphicSpecularColor=[0.5 0.5 0.5 1.0]  GraphicAmbientColor=[0.15 0.15 0.15 1.0]  GraphicEmissiveColor=[0.0 0.0 0.0 1.0]  GraphicShininess=75  GraphicOpacity=1.0  GeometryShape=FromFile  RectangleSize=[1 1]  RectangleSizeUnits=m  BrickDimensions=[1 1 1]  BrickDimensionUnits=mm  CylinderRadius=1  CylinderRadiusUnits=m  CylinderLength=1  CylinderLengthUnits=m  SphereRadius=1  SphereRadiusUnits=m  EllipsoidRadii=[1 1 1]  EllipsoidRadiiUnits=m  ExtrusionCrossSection=[1 1; -1 1; -1 -1; 1 -1]  ExtrusionCrossSectionUnits=m  ExtrusionLength=1  ExtrusionLengthUnits=m  PolygonNumSides=3  PolygonOuterRadius=1  PolygonOuterRadiusUnits=m  ExtGeomFileType=STL  ExtGeomFileName=D:\Ker Lann\systemes\darwin\kinematics\STL\Right_Arm.STL  ExtGeomFileUnits=mm  RevolutionCrossSection=[1 1; 1 -1; 2 -1; 2 1]  RevolutionCrossSectionUnits=m  RevolutionExtent=Full  RevolutionAngle=180  RevolutionAngleUnits=deg  BlockFunction=simmechanics.library.body_elements.solid
  Right Shoulder Roll : PMIOPort  Port=1  Side=Left
  Right Elbow : PMIOPort  Port=2  Side=Right
  connections:
  Right Arm Axis to Right Forearm Base/LConn1 -- Right Shoulder Roll/RConn1 -- Solid/RConn1
  Right Arm Axis to Right Forearm Base/RConn1 -- Right Elbow/RConn1

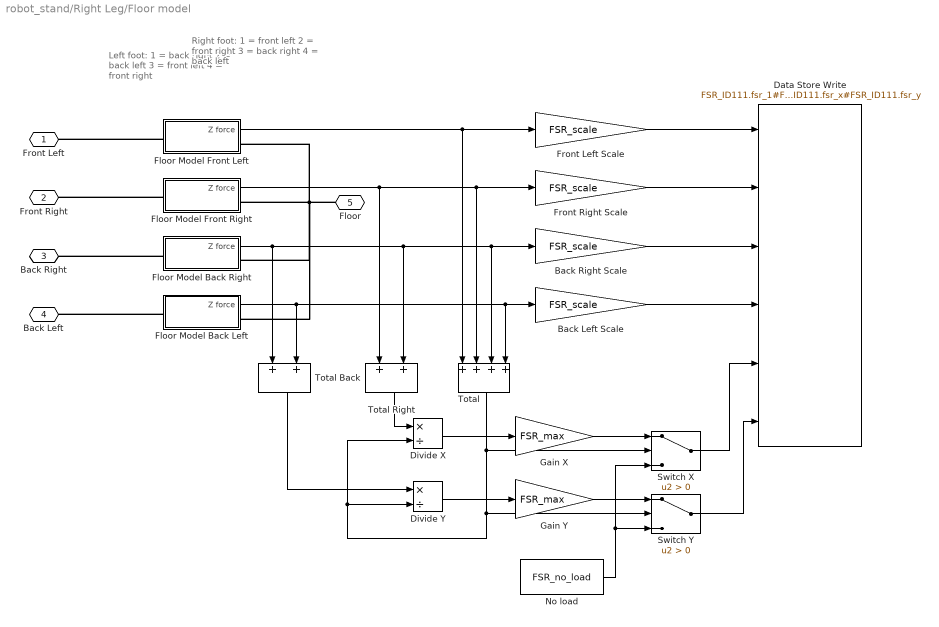
== system robot_stand/Right Leg/Floor model ==
  note: Left foot:
      | 1 = back right
      | 2 = back left
      | 3 = front left
      | 4 = front right
  note: Right foot:
      | 1 = front left
      | 2 = front right
      | 3 = back right
      | 4 = back left
  Back Left Scale : Gain  Gain=FSR_scale  OutDataTypeStr=uint16  SampleTime=FSR_sample_time  SaturateOnIntegerOverflow=on
  Back Right Scale : Gain  Gain=FSR_scale  OutDataTypeStr=uint16  SampleTime=FSR_sample_time  SaturateOnIntegerOverflow=on
  Data Store Write : DataStoreWrite  DataStoreName=FSR_ID111  DataStoreElements=FSR_ID111.fsr_1#FSR_ID111.fsr_2#FSR_ID111.fsr_3#FSR_ID111.fsr_4#FSR_ID111.fsr_x#FSR_ID111.fsr_y
  Divide X : Product  Inputs=*/
  Divide Y : Product  Inputs=*/
  Floor Model Back Left : Subsystem
  Floor Model Back Right : Subsystem
  Floor Model Front Left : Subsystem
  Floor Model Front Right : Subsystem
  Front Left Scale : Gain  Gain=FSR_scale  OutDataTypeStr=uint16  SampleTime=FSR_sample_time  SaturateOnIntegerOverflow=on
  Front Right Scale : Gain  Gain=FSR_scale  OutDataTypeStr=uint16  SampleTime=FSR_sample_time  SaturateOnIntegerOverflow=on
  Gain X : Gain  Gain=FSR_max  OutDataTypeStr=uint8  SaturateOnIntegerOverflow=on
  Gain Y : Gain  Gain=FSR_max  OutDataTypeStr=uint8  SaturateOnIntegerOverflow=on
  No load : Constant  Value=FSR_no_load  OutDataTypeStr=uint8
  Switch X : Switch  Criteria=u2 > Threshold
  Switch Y : Switch  Criteria=u2 > Threshold
  Total : Sum  Inputs=++++  SampleTime=FSR_sample_time
  Total Back : Sum  SampleTime=FSR_sample_time
  Total Right : Sum  SampleTime=FSR_sample_time
  Front Left : PMIOPort  Port=1  Side=Left
  Front Right : PMIOPort  Port=2  Side=Left
  Back Right : PMIOPort  Port=3  Side=Left
  Back Left : PMIOPort  Port=4  Side=Left
  Floor : PMIOPort  Port=5  Side=Right
  wires:
  Floor Model Front Left/1(Z force) -> Total/1, Front Left Scale/1
  Floor Model Front Right/1(Z force) -> Total Right/1, Front Right Scale/1, Total/2
  Floor Model Back Right/1(Z force) -> Total Back/1, Total/3, Back Right Scale/1, Total Right/2
  Floor Model Back Left/1(Z force) -> Total Back/2, Total/4, Back Left Scale/1
  Total/1 -> Divide Y/2, Divide X/2, Switch Y/2, Switch X/2
  No load/1 -> Switch Y/3, Switch X/3
  Divide X/1 -> Gain X/1
  Total Right/1 -> Divide X/1
  Divide Y/1 -> Gain Y/1
  Total Back/1 -> Divide Y/1
  Gain X/1 -> Switch X/1
  Gain Y/1 -> Switch Y/1
  Switch X/1 -> Data Store Write/5
  Switch Y/1 -> Data Store Write/6
  Front Left Scale/1 -> Data Store Write/1
  Front Right Scale/1 -> Data Store Write/2
  Back Right Scale/1 -> Data Store Write/3
  Back Left Scale/1 -> Data Store Write/4
  connections:
  Floor Model Back Left/LConn1 -- Back Left/RConn1
  Floor Model Back Right/LConn1 -- Back Right/RConn1
  Floor Model Front Right/LConn1 -- Front Right/RConn1
  Floor Model Front Left/LConn1 -- Front Left/RConn1
  Floor/RConn1 -- Floor Model Front Left/RConn1 -- Floor Model Front Right/RConn1 -- Floor Model Back Right/RConn1 -- Floor Model Back Left/RConn1

== system robot_stand/Right Leg/Right Ankle ==
  Right Ankle Base to Right Foot Base : sm_lib/Frames and Transforms/Rigid Transform  TranslationMethod=Cartesian  TranslationLengthUnit=mm  TranslationStandardAxis=+Z  TranslationStandardOffset=0  TranslationCartesianOffset=[-19.35 0 -24]  TranslationROffset=0  TranslationROffsetUnits=m  TranslationZOffset=0  TranslationZOffsetUnits=m  TranslationThetaOffset=0  TranslationThetaOffsetUnits=deg  RotationMethod=AlignedAxes  RotationAngleUnits=deg  RotationStandardAxis=+Z  RotationAngle=0  RotationArbitraryAxis=[0 0 1]  FollAlignAxisA=+X  BaseAlignAxisA=+Z  FollAlignAxisB=+Y  BaseAlignAxisB=-Y  RotationMatrix=[1 0 0; 0 1 0; 0 0 1]  BlockFunction=simmechanics.library.frames_transforms.rigid_transform
  Solid : sm_lib/Body Elements/Solid  InertiaType=Custom  Mass=166.79  MassUnits=g  CenterOfMass=[-18.06 -11.21 -24.20]  CenterOfMassUnits=mm  MomentsOfInertia=[6948 12212 11817]  MomentsOfInertiaUnits=g*mm^2  ProductsOfInertia=[-194 117 4006]  ProductsOfInertiaUnits=g*mm^2  DensityBased=on  Density=1000  DensityUnits=kg/(m^3)  GraphicType=FromGeometry  MarkerShape=Sphere  MarkerSize=10  MarkerSizeUnits=m  GraphicVisPropType=SimpleVisualProperties  GraphicDiffuseColor=[0.5 0.5 0.5]  GraphicSpecularColor=[0.5 0.5 0.5 1.0]  GraphicAmbientColor=[0.15 0.15 0.15 1.0]  GraphicEmissiveColor=[0.0 0.0 0.0 1.0]  GraphicShininess=75  GraphicOpacity=1.0  GeometryShape=FromFile  RectangleSize=[1 1]  RectangleSizeUnits=m  BrickDimensions=[1 1 1]  BrickDimensionUnits=m  CylinderRadius=1  CylinderRadiusUnits=m  CylinderLength=1  CylinderLengthUnits=m  SphereRadius=1  SphereRadiusUnits=m  EllipsoidRadii=[1 1 1]  EllipsoidRadiiUnits=m  ExtrusionCrossSection=[1 1; -1 1; -1 -1; 1 -1]  ExtrusionCrossSectionUnits=m  ExtrusionLength=1  ExtrusionLengthUnits=m  PolygonNumSides=3  PolygonOuterRadius=1  PolygonOuterRadiusUnits=m  ExtGeomFileType=STL  ExtGeomFileName=D:\Ker Lann\systemes\darwin\kinematics\STL\Right_Ankle.STL  ExtGeomFileUnits=mm  RevolutionCrossSection=[1 1; 1 -1; 2 -1; 2 1]  RevolutionCrossSectionUnits=m  RevolutionExtent=Full  RevolutionAngle=180  RevolutionAngleUnits=deg  BlockFunction=simmechanics.library.body_elements.solid
  Right Ankle Pitch : PMIOPort  Port=1  Side=Left
  Right Ankle Roll : PMIOPort  Port=2  Side=Right
  connections:
  Solid/RConn1 -- Right Ankle Base to Right Foot Base/LConn1 -- Right Ankle Pitch/RConn1
  Right Ankle Roll/RConn1 -- Right Ankle Base to Right Foot Base/RConn1
